simulink model "prac2"  (R2022b)
settings: Solver=VariableStepAuto  StartTime=0.0  StopTime=100  RelTol=1e-3
settings Model: Creator=ESTHER  LastModifiedBy=ESTHER

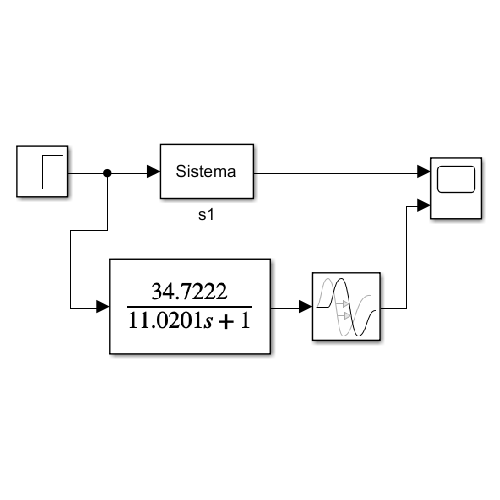
[thumbnail: Simulink's stored preview of the top-level diagram]
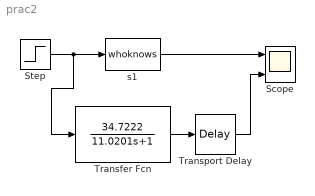
== system prac2 ==
  Scope : Scope  NumInputPorts=2
  Step : Step  SampleTime=0
  Transfer Fcn : TransferFcn  Numerator=[34.7222]  Denominator=[11.0201 1]
  Transport Delay : TransportDelay
  s1 : M-S-Function  FunctionName=whoknows  Parameters=L, P1, P2, T, R  mask{L=6, P1=1, P2=3, T=2, R=0}
      mask prompts: L "Laboratorio"; P1 "Primer digito del Puesto"; P2 "Segundo digito del Puesto"; T "Tipo de Planta"; R "Ruido"
      mask Display: disp('Sistema')
  wires:
  s1/1 -> Scope/1
  Step/1 -> Transfer Fcn/1, s1/1
  Transfer Fcn/1 -> Transport Delay/1
  Transport Delay/1 -> Scope/2
